simulink model "pendulum"  (R2015b)
settings: Solver=VariableStepAuto  StartTime=0.0  StopTime=5  RelTol=1e-3
settings Model: Creator=Andreas  LastModifiedBy=Andreas

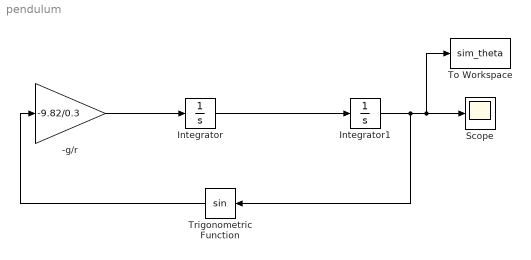
== system pendulum ==
  -g/r : Gain  Gain=-9.82/0.3
  Integrator : Integrator  InitialCondition=1
  Integrator1 : Integrator
  Scope : Scope
  To Workspace : ToWorkspace  VariableName=sim_theta  SaveFormat=Timeseries  SampleTime=-1
  Trigonometric Function : Trigonometry
  wires:
  Integrator/1 -> Integrator1/1
  -g/r/1 -> Integrator/1
  Integrator1/1 -> Trigonometric Function/1, To Workspace/1, Scope/1
  Trigonometric Function/1 -> -g/r/1
